simulink model "syt_a22"  (Simulink 7.0)
settings: Solver=ode45  StartTime=0.0  StopTime=10.0  RelTol=1e-3
values from neighbouring files (symbols this model uses):
  C = T/R    (= 0.001)    [syt_aufg13.m]    (also in syt_aufg8.m)
  R = 10000    [syt_aufg13.m]    (also in syt_aufg8.m = 1000)
settings Model: Creator=LAT04  LastModifiedBy=LAT04

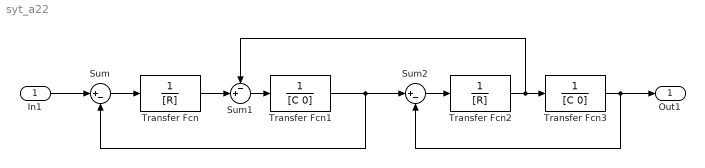
== system syt_a22 ==
  In1 : Inport  OutDataType=sfix(16)  OutScaling=2^0
  Sum : Sum  Inputs=|+-  OutDataType=sfix(16)  OutScaling=2^0
  Sum1 : Sum  Inputs=-+|  OutDataType=sfix(16)  OutScaling=2^0
  Sum2 : Sum  Inputs=|+-  OutDataType=sfix(16)  OutScaling=2^0
  Transfer Fcn : TransferFcn  Denominator=[R]
  Transfer Fcn1 : TransferFcn  Denominator=[C 0]
  Transfer Fcn2 : TransferFcn  Denominator=[R]
  Transfer Fcn3 : TransferFcn  Denominator=[C 0]
  Out1 : Outport  OutDataType=sfix(16)  OutScaling=2^0
  wires:
  In1/1 -> Sum/1
  Sum/1 -> Transfer Fcn/1
  Transfer Fcn/1 -> Sum1/2
  Sum1/1 -> Transfer Fcn1/1
  Transfer Fcn1/1 -> Sum2/1, Sum/2
  Sum2/1 -> Transfer Fcn2/1
  Transfer Fcn2/1 -> Transfer Fcn3/1, Sum1/1
  Transfer Fcn3/1 -> Out1/1, Sum2/2
